simulink model "mono_camera_lane_tracking_with_ros"  (R2019b)
settings: Solver=FixedStepDiscrete  StartTime=0.0  StopTime=inf  FixedStep=Ts  RelTol=1e-3
undefined symbols (not defined in the file): PredictionHorizon, Ts
libraries: robotlib x17, mpcadaslib x1
settings Model: Creator=The MathWorks, Inc.  LastModifiedBy=senoa95
settings DataIOCC: SaveOutput=off  SaveTime=off  ReturnWorkspaceOutputs=off
settings OptimizationCC: DefaultParameterBehavior=Inlined  UseDivisionForNetSlopeComputation=on  GainParamInheritBuiltInType=on  UseFloatMulNetSlope=on  DefaultUnderspecifiedDataType=single  InlineInvariantSignals=on  PassReuseOutputArgsAs=Individual arguments  ZeroExternalMemoryAtStartup=off  ZeroInternalMemoryAtStartup=off  NoFixptDivByZeroProtection=on  EfficientFloat2IntCast=on  LifeSpan=1  OptimizeBlockOrder=speed  DifferentSizesBufferReuse=on  EfficientTunableParamExpr=on
settings DebuggingCC: ParameterPrecisionLossMsg=none  ParameterTunabilityLossMsg=error  PregeneratedLibrarySubsystemCodeDiagnostic=none  ArithmeticOperatorsInVariantConditions=warning
settings HardwareCC: ProdBitPerLong=64  ProdLongLongMode=on  ProdHWDeviceType=Intel->x86-64 (Linux 64)
settings SFSimCC: SimUseLocalCustomCode=off  MATLABDynamicMemAlloc=off
settings RTWCC: SystemTargetFile=ert.tlc  TemplateMakefile=ert_default_tmf  GenerateReport=on  RTWUseLocalCustomCode=off  BuildConfiguration=Faster Runs  IncludeHyperlinkInReport=on  LaunchReport=on  TargetLang=C++  GenerateTraceInfo=on  GenerateTraceReport=on  GenerateTraceReportSl=on  GenerateTraceReportSf=on  GenerateTraceReportEml=on
settings CodeAppCC: ForceParamTrailComments=on  IgnoreCustomStorageClasses=off  MaxIdLength=63  OperatorAnnotations=on  SimulinkDataObjDesc=on  SFDataObjDesc=on  CustomSymbolStrGlobalVar=rt$N$M  CustomSymbolStrType=$N$M  CustomSymbolStrFcn=$N$M$F  CustomSymbolStrMacro=$N$M  InsertBlockDesc=on
settings ERTTargetCC: TargetLangStandard=C++03 (ISO)  GenerateSampleERTMain=on  IncludeMdlTerminateFcn=off  CombineSignalStateStructs=on  SupportAbsoluteTime=off  MultiInstanceERTCode=on  CodeInterfacePackaging=C++ class  SupportComplex=off  SupportNonInlinedSFcns=on  InlinedParameterPlacement=NonHierarchical  RootIOFormat=Structure reference  ERTCustomFileTemplate=example_file_process.tlc

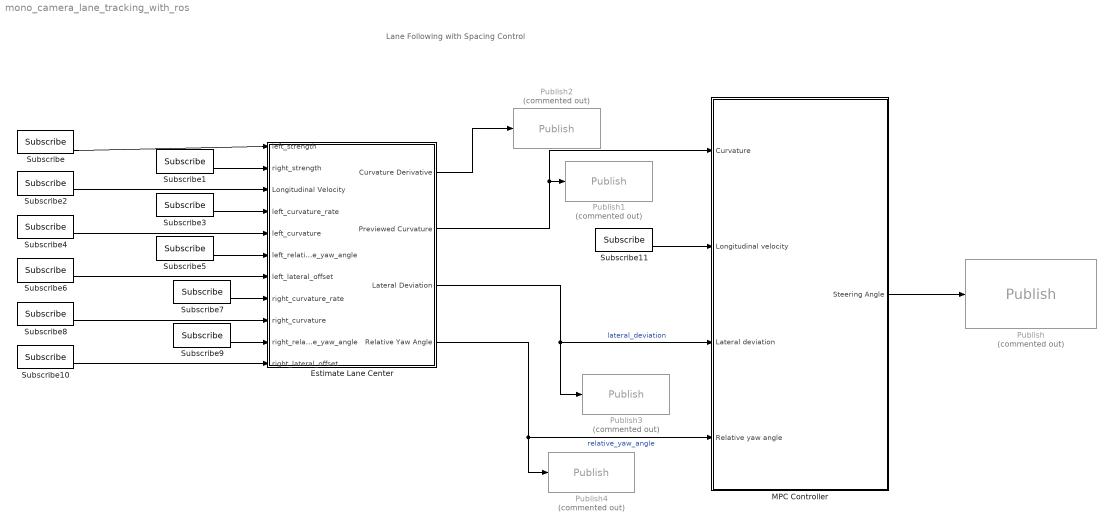
== system mono_camera_lane_tracking_with_ros ==
  note: Lane Following with Spacing Control
  Estimate Lane Center : Subsystem  TreatAsAtomicUnit=on  VariantControl=v2
      settings: RTWFileNameOpts=Use function name
  "MPC Controller " : Subsystem
  Publish : robotlib/Publish  Commented=on  topicSource=Specify your own  topic=/steering_angle  messageType=geometry_msgs/Point  messageQueueLength=1
      settings: SourceProductName=ROS Toolbox
  Publish1 : robotlib/Publish  Commented=on  topicSource=Specify your own  topic=/lane/center/curvature  messageType=std_msgs/Int32  messageQueueLength=1
      settings: SourceProductName=ROS Toolbox
  Publish2 : robotlib/Publish  Commented=on  topicSource=Specify your own  topic=/lane/center/curvature_derivative  messageType=std_msgs/Int32  messageQueueLength=1
      settings: SourceProductName=ROS Toolbox
  Publish3 : robotlib/Publish  Commented=on  topicSource=Specify your own  topic=/lane/center/lateral_deviation  messageType=std_msgs/Int32  messageQueueLength=1
      settings: SourceProductName=ROS Toolbox
  Publish4 : robotlib/Publish  Commented=on  topicSource=Specify your own  topic=/lane/center/lateral_deviation  messageType=std_msgs/Int32  messageQueueLength=1
      settings: SourceProductName=ROS Toolbox
  Subscribe : robotlib/Subscribe  topicSource=Specify your own  topic=/lanes/left/strength  messageType=std_msgs/Int32  sampleTime=-1  messageQueueLength=1
      settings: SourceProductName=ROS Toolbox
  Subscribe1 : robotlib/Subscribe  topicSource=Specify your own  topic=/lanes/left/strength  messageType=std_msgs/Int32  sampleTime=-1  messageQueueLength=1
      settings: SourceProductName=ROS Toolbox
  Subscribe10 : robotlib/Subscribe  topicSource=Specify your own  topic=/lanes/right/lateral_offset  messageType=std_msgs/Int32  sampleTime=-1  messageQueueLength=1
      settings: SourceProductName=ROS Toolbox
  Subscribe11 : robotlib/Subscribe  topicSource=Specify your own  topic=/turtle_velocity  messageType=std_msgs/Int32  sampleTime=-1  messageQueueLength=1
      settings: SourceProductName=ROS Toolbox
  Subscribe2 : robotlib/Subscribe  topicSource=Specify your own  topic=/turtle_velocity  messageType=std_msgs/Int32  sampleTime=-1  messageQueueLength=1
      settings: SourceProductName=ROS Toolbox
  Subscribe3 : robotlib/Subscribe  topicSource=Specify your own  topic=/lanes/left/curvature_rate  messageType=std_msgs/Int32  sampleTime=-1  messageQueueLength=1
      settings: SourceProductName=ROS Toolbox
  Subscribe4 : robotlib/Subscribe  topicSource=Specify your own  topic=/lanes/left/curvature  messageType=std_msgs/Int32  sampleTime=-1  messageQueueLength=1
      settings: SourceProductName=ROS Toolbox
  Subscribe5 : robotlib/Subscribe  topicSource=Specify your own  topic=/lanes/left/relative_yaw_angle  messageType=std_msgs/Int32  sampleTime=-1  messageQueueLength=1
      settings: SourceProductName=ROS Toolbox
  Subscribe6 : robotlib/Subscribe  topicSource=Specify your own  topic=/lanes/left/lateral_offset  messageType=std_msgs/Int32  sampleTime=-1  messageQueueLength=1
      settings: SourceProductName=ROS Toolbox
  Subscribe7 : robotlib/Subscribe  topicSource=Specify your own  topic=/lanes/right/curvature_rate  messageType=std_msgs/Int32  sampleTime=-1  messageQueueLength=1
      settings: SourceProductName=ROS Toolbox
  Subscribe8 : robotlib/Subscribe  topicSource=Specify your own  topic=/lanes/right/curvature  messageType=std_msgs/Int32  sampleTime=-1  messageQueueLength=1
      settings: SourceProductName=ROS Toolbox
  Subscribe9 : robotlib/Subscribe  topicSource=Specify your own  topic=/lanes/right/relative_yaw_angle  messageType=std_msgs/Int32  sampleTime=-1  messageQueueLength=1
      settings: SourceProductName=ROS Toolbox
  wires:
  Subscribe11/2 -> "MPC Controller "/2(Longitudinal velocity)
  Estimate Lane Center/2(Previewed Curvature) -> "MPC Controller "/1(Curvature), Publish1/1
  "MPC Controller "/1(Steering Angle) -> Publish/1
  Estimate Lane Center/3(Lateral Deviation) -> Publish3/1, "MPC Controller "/3(Lateral deviation)  "lateral_deviation"
  Estimate Lane Center/4(Relative Yaw Angle) -> Publish4/1, "MPC Controller "/4(Relative yaw angle)  "relative_yaw_angle"
  Subscribe2/2 -> Estimate Lane Center/3(Longitudinal Velocity)
  Subscribe/2 -> Estimate Lane Center/1(left_strength)
  Subscribe1/2 -> Estimate Lane Center/2(right_strength)
  Subscribe3/2 -> Estimate Lane Center/4(left_curvature_rate)
  Subscribe4/2 -> Estimate Lane Center/5(left_curvature)
  Subscribe6/2 -> Estimate Lane Center/7(left_lateral_offset)
  Subscribe5/2 -> Estimate Lane Center/6(left_relative_yaw_angle)
  Subscribe7/2 -> Estimate Lane Center/8(right_curvature_rate)
  Subscribe8/2 -> Estimate Lane Center/9(right_curvature)
  Subscribe9/2 -> Estimate Lane Center/10(right_relative_yaw_angle)
  Subscribe10/2 -> Estimate Lane Center/11(right_lateral_offset)
  Estimate Lane Center/1(Curvature Derivative) -> Publish2/1

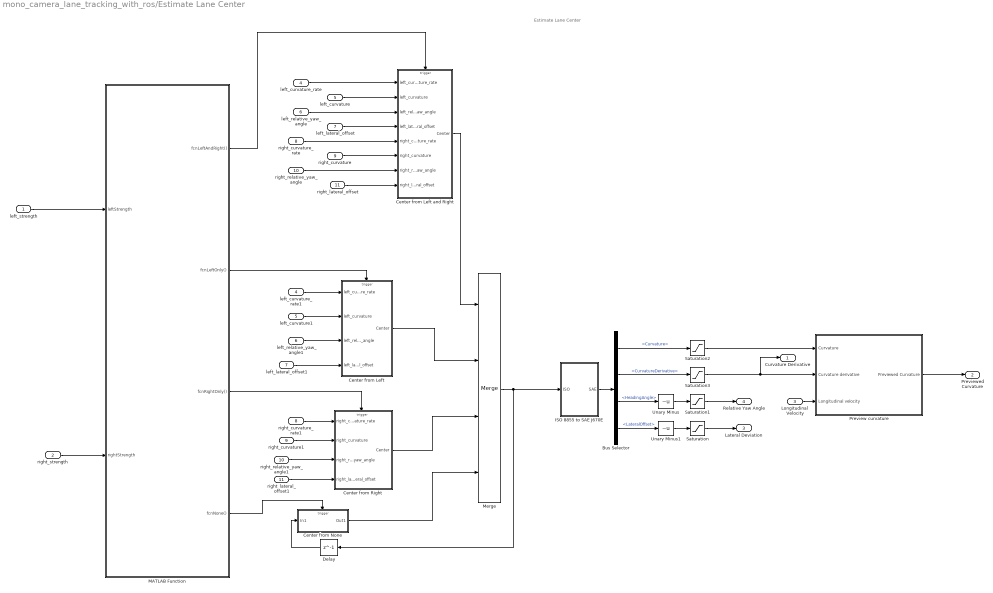
== system mono_camera_lane_tracking_with_ros/Estimate Lane Center ==
  note: Estimate Lane Center
  left_strength : Inport
  right_strength : Inport  Port=2
  Longitudinal Velocity : Inport  Port=3
  left_curvature_rate : Inport  Port=4
  left_curvature : Inport  Port=5
  left_relative_yaw_angle : Inport  Port=6
  left_lateral_offset : Inport  Port=7
  right_curvature_rate : Inport  Port=8
  right_curvature : Inport  Port=9
  right_relative_yaw_angle : Inport  Port=10
  right_lateral_offset : Inport  Port=11
  Bus Selector : BusSelector  OutputSignals=Curvature,CurvatureDerivative,HeadingAngle,LateralOffset
  Center from Left : Subsystem  TreatAsAtomicUnit=on
  Center from Left and Right : Subsystem  TreatAsAtomicUnit=on
  Center from None : Subsystem  TreatAsAtomicUnit=on
  Center from Right : Subsystem  TreatAsAtomicUnit=on
  Delay : Delay  DelayLength=1
  ISO 8855 to SAE J670E : Subsystem
  MATLAB Function : MATLAB Function  TreatAsAtomicUnit=on
  Merge : Merge  Inputs=4
  Preview curvature : Subsystem
  Saturation : Saturate
  Saturation1 : Saturate  UpperLimit=0.6  LowerLimit=-0.6
  Saturation2 : Saturate  UpperLimit=0.15  LowerLimit=-0.15
  Saturation3 : Saturate  UpperLimit=0.06  LowerLimit=-0.06
  Unary Minus : UnaryMinus
  Unary Minus1 : UnaryMinus
  left_curvature1 : InportShadow  Port=5
  left_curvature_rate1 : InportShadow  Port=4
  left_lateral_offset1 : InportShadow  Port=7
  left_relative_yaw_angle1 : InportShadow  Port=6
  right_curvature1 : InportShadow  Port=9
  right_curvature_rate1 : InportShadow  Port=8
  right_lateral_offset1 : InportShadow  Port=11
  right_relative_yaw_angle1 : InportShadow  Port=10
  Curvature Derivative : Outport  OutDataTypeStr=int32
  Previewed Curvature : Outport  Port=2  OutDataTypeStr=int32  VectorParamsAs1DForOutWhenUnconnected=off
  Lateral Deviation : Outport  Port=3  OutDataTypeStr=int32  VectorParamsAs1DForOutWhenUnconnected=off
  Relative Yaw Angle : Outport  Port=4  OutDataTypeStr=int32  VectorParamsAs1DForOutWhenUnconnected=off
  wires:
  Center from Right/1(Center) -> Merge/3
  MATLAB Function/2(fcnLeftOnly()) -> Center from Left/Trigger
  Center from None/1(Out1) -> Merge/4
  MATLAB Function/1(fcnLeftAndRight()) -> Center from Left and Right/Trigger
  Delay/1 -> Center from None/1(In1)
  Center from Left and Right/1(Center) -> Merge/1
  MATLAB Function/3(fcnRightOnly()) -> Center from Right/Trigger
  MATLAB Function/4(fcnNone()) -> Center from None/Trigger
  Center from Left/1(Center) -> Merge/2
  Merge/1 -> ISO 8855 to SAE J670E/1(ISO), Delay/1
  Saturation3/1 -> Curvature Derivative/1, Preview curvature/2(Curvature derivative)
  Saturation2/1 -> Preview curvature/1(Curvature)
  Saturation1/1 -> Relative Yaw Angle/1
  Saturation/1 -> Lateral Deviation/1
  Unary Minus/1 -> Saturation1/1
  Preview curvature/1(Previewed Curvature) -> Previewed Curvature/1
  Longitudinal Velocity/1 -> Preview curvature/3(Longitudinal velocity)
  Bus Selector/2 -> Saturation3/1  "<CurvatureDerivative>"
  Bus Selector/1 -> Saturation2/1  "<Curvature>"
  Unary Minus1/1 -> Saturation/1
  Bus Selector/4 -> Unary Minus1/1  "<LateralOffset>"
  Bus Selector/3 -> Unary Minus/1  "<HeadingAngle>"
  ISO 8855 to SAE J670E/1(SAE) -> Bus Selector/1
  left_strength/1 -> MATLAB Function/1(leftStrength)
  right_strength/1 -> MATLAB Function/2(rightStrength)
  left_curvature_rate/1 -> Center from Left and Right/1(left_curvature_rate)
  right_relative_yaw_angle/1 -> Center from Left and Right/7(right_relative_yaw_angle)
  right_lateral_offset/1 -> Center from Left and Right/8(right_lateral_offset)
  left_lateral_offset/1 -> Center from Left and Right/4(left_lateral_offset)
  left_curvature/1 -> Center from Left and Right/2(left_curvature)
  left_relative_yaw_angle/1 -> Center from Left and Right/3(left_relative_yaw_angle)
  right_curvature_rate/1 -> Center from Left and Right/5(right_curvature_rate)
  right_curvature/1 -> Center from Left and Right/6(right_curvature)
  left_curvature_rate1/1 -> Center from Left/1(left_curvature_rate)
  left_curvature1/1 -> Center from Left/2(left_curvature)
  left_relative_yaw_angle1/1 -> Center from Left/3(left_relative_yaw_angle)
  left_lateral_offset1/1 -> Center from Left/4(left_lateral_offset)
  right_curvature_rate1/1 -> Center from Right/1(right_curvature_rate)
  right_curvature1/1 -> Center from Right/2(right_curvature)
  right_relative_yaw_angle1/1 -> Center from Right/3(right_relative_yaw_angle)
  right_lateral_offset1/1 -> Center from Right/4(right_lateral_offset)

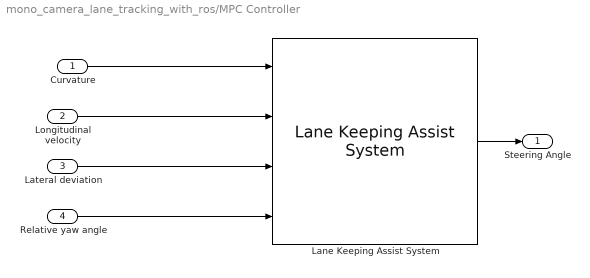
== system mono_camera_lane_tracking_with_ros/MPC Controller  ==
  Curvature : Inport
  Longitudinal velocity : Inport  Port=2
  Lateral deviation : Inport  Port=3
  Relative yaw angle : Inport  Port=4
  Lane Keeping Assist System : mpcadaslib/Lane Keeping Assist System  ModelType=Use vehicle parameters  VehicleMass=1575  VehicleYawInertia=2875  LengthToFront=1.2  LengthToRear=1.6  FrontTireStiffness=19000  RearTireStiffness=33000  EgoModelMatrixA=[-4.4021 ,-12.4603;1.3913,-5.1868]  EgoModelMatrixB=[24.1270;15.8609]  EgoModelMatrixC=[1,0;0,1]  InitialLongVel=15  TransportLag=0  MinSteering=-0.26  umin_ext=off  MaxSteering=0.26  umax_ext=off  Ts=0.1  PredictionHorizon=10  ControllerBehavior=0.5  suboptimal=off  maxiter=10  datatypeopt=double  optmode=off  trackmode=off
      settings: SourceProductName=Model Predictive Control Toolbox  SourceProductBaseCode=MP
  Steering Angle : Outport  OutDataTypeStr=int32  VectorParamsAs1DForOutWhenUnconnected=off
  wires:
  Lane Keeping Assist System/1 -> Steering Angle/1
  Curvature/1 -> Lane Keeping Assist System/1
  Longitudinal velocity/1 -> Lane Keeping Assist System/2
  Lateral deviation/1 -> Lane Keeping Assist System/3
  Relative yaw angle/1 -> Lane Keeping Assist System/4

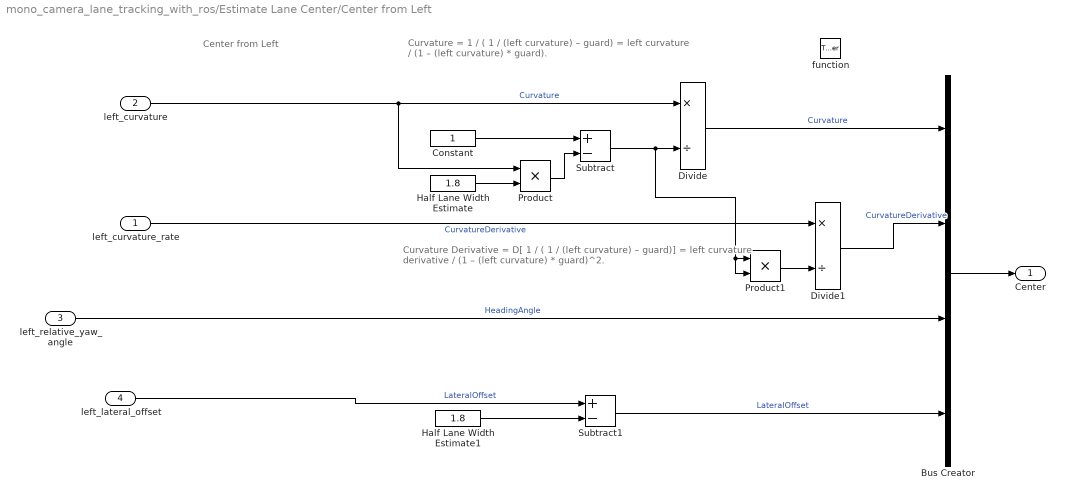
== system mono_camera_lane_tracking_with_ros/Estimate Lane Center/Center from Left ==
  note: Curvature Derivative
      | = D[ 1 / ( 1 / (left curvature) – guard)]
      | = left curvature derivative / (1 – (left curvature) * guard)^2.
  note: Center from Left
  note: Curvature
      | = 1 / ( 1 / (left curvature) – guard)
      | = left curvature / (1 – (left curvature) * guard).
  left_curvature_rate : Inport
  left_curvature : Inport  Port=2
  left_relative_yaw_angle : Inport  Port=3
  left_lateral_offset : Inport  Port=4
  function : TriggerPort  TriggerType=function-call  VariantControl=Variant
  Bus Creator : BusCreator  Inputs=4
  Constant : Constant  OutDataTypeStr=Inherit: Inherit via back propagation
  Divide : Product  Inputs=*/
  Divide1 : Product  Inputs=*/
  Half Lane Width Estimate : Constant  Value=1.8  OutDataTypeStr=Inherit: Inherit via back propagation
  Half Lane Width Estimate1 : Constant  Value=1.8  OutDataTypeStr=Inherit: Inherit via back propagation
  Product : Product
  Product1 : Product
  Subtract : Sum  Inputs=+-
  Subtract1 : Sum  Inputs=+-
  Center : Outport  VectorParamsAs1DForOutWhenUnconnected=off
  wires:
  Product/1 -> Subtract/2
  Half Lane Width Estimate1/1 -> Subtract1/2
  left_lateral_offset/1 -> Subtract1/1  "LateralOffset"
  Product1/1 -> Divide1/2
  left_curvature_rate/1 -> Divide1/1  "CurvatureDerivative"
  Constant/1 -> Subtract/1
  Half Lane Width Estimate/1 -> Product/2
  Subtract/1 -> Divide/2, Product1/1, Product1/2
  left_curvature/1 -> Divide/1, Product/1  "Curvature"
  Subtract1/1 -> Bus Creator/4  "LateralOffset"
  left_relative_yaw_angle/1 -> Bus Creator/3  "HeadingAngle"
  Divide/1 -> Bus Creator/1  "Curvature"
  Divide1/1 -> Bus Creator/2  "CurvatureDerivative"
  Bus Creator/1 -> Center/1

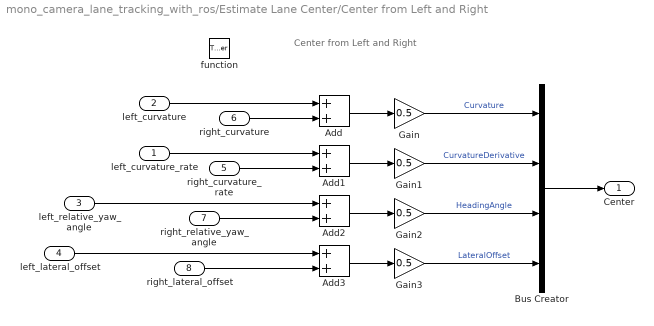
== system mono_camera_lane_tracking_with_ros/Estimate Lane Center/Center from Left and Right ==
  note: Center from Left and Right
  left_curvature_rate : Inport
  left_curvature : Inport  Port=2
  left_relative_yaw_angle : Inport  Port=3
  left_lateral_offset : Inport  Port=4
  right_curvature_rate : Inport  Port=5
  right_curvature : Inport  Port=6
  right_relative_yaw_angle : Inport  Port=7
  right_lateral_offset : Inport  Port=8
  function : TriggerPort  TriggerType=function-call  VariantControl=Variant
  Add{,1..3} (4 alike) : Sum
  Bus Creator : BusCreator  Inputs=4
  Gain{,1..3} (4 alike) : Gain  Gain=0.5
  Center : Outport  VectorParamsAs1DForOutWhenUnconnected=off
  wires:
  left_lateral_offset/1 -> Add3/1
  right_lateral_offset/1 -> Add3/2
  right_relative_yaw_angle/1 -> Add2/2
  left_relative_yaw_angle/1 -> Add2/1
  right_curvature_rate/1 -> Add1/2
  left_curvature_rate/1 -> Add1/1
  left_curvature/1 -> Add/1
  Bus Creator/1 -> Center/1
  Gain3/1 -> Bus Creator/4  "LateralOffset"
  Add3/1 -> Gain3/1
  Gain2/1 -> Bus Creator/3  "HeadingAngle"
  Add2/1 -> Gain2/1
  Gain1/1 -> Bus Creator/2  "CurvatureDerivative"
  Add1/1 -> Gain1/1
  Gain/1 -> Bus Creator/1  "Curvature"
  Add/1 -> Gain/1
  right_curvature/1 -> Add/2

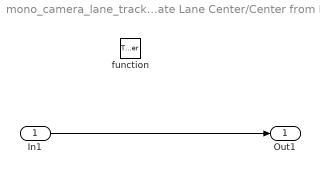
== system mono_camera_lane_tracking_with_ros/Estimate Lane Center/Center from None ==
  In1 : Inport
  function : TriggerPort  TriggerType=function-call  VariantControl=Variant
  Out1 : Outport  VectorParamsAs1DForOutWhenUnconnected=off
  wires:
  In1/1 -> Out1/1

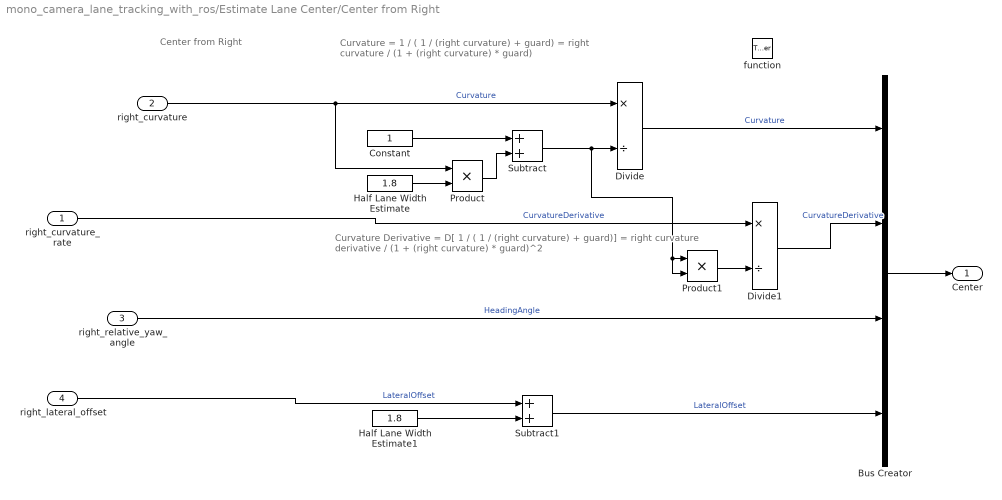
== system mono_camera_lane_tracking_with_ros/Estimate Lane Center/Center from Right ==
  note: Curvature Derivative
      | = D[ 1 / ( 1 / (right curvature) + guard)]
      | = right curvature derivative / (1 + (right curvature) * guard)^2
  note: Curvature
      | = 1 / ( 1 / (right curvature) + guard)
      | = right curvature / (1 + (right curvature) * guard)
  note: Center from Right
  right_curvature_rate : Inport
  right_curvature : Inport  Port=2
  right_relative_yaw_angle : Inport  Port=3
  right_lateral_offset : Inport  Port=4
  function : TriggerPort  TriggerType=function-call  VariantControl=Variant
  Bus Creator : BusCreator  Inputs=4
  Constant : Constant  OutDataTypeStr=Inherit: Inherit via back propagation
  Divide : Product  Inputs=*/
  Divide1 : Product  Inputs=*/
  Half Lane Width Estimate : Constant  Value=1.8  OutDataTypeStr=Inherit: Inherit via back propagation
  Half Lane Width Estimate1 : Constant  Value=1.8  OutDataTypeStr=Inherit: Inherit via back propagation
  Product : Product
  Product1 : Product
  Subtract : Sum
  Subtract1 : Sum
  Center : Outport  VectorParamsAs1DForOutWhenUnconnected=off
  wires:
  Half Lane Width Estimate/1 -> Product/2
  Product/1 -> Subtract/2
  Constant/1 -> Subtract/1
  Subtract/1 -> Divide/2, Product1/1, Product1/2
  right_curvature/1 -> Divide/1, Product/1  "Curvature"
  Bus Creator/1 -> Center/1
  Subtract1/1 -> Bus Creator/4  "LateralOffset"
  Divide/1 -> Bus Creator/1  "Curvature"
  right_lateral_offset/1 -> Subtract1/1  "LateralOffset"
  Half Lane Width Estimate1/1 -> Subtract1/2
  right_relative_yaw_angle/1 -> Bus Creator/3  "HeadingAngle"
  Product1/1 -> Divide1/2
  Divide1/1 -> Bus Creator/2  "CurvatureDerivative"
  right_curvature_rate/1 -> Divide1/1  "CurvatureDerivative"

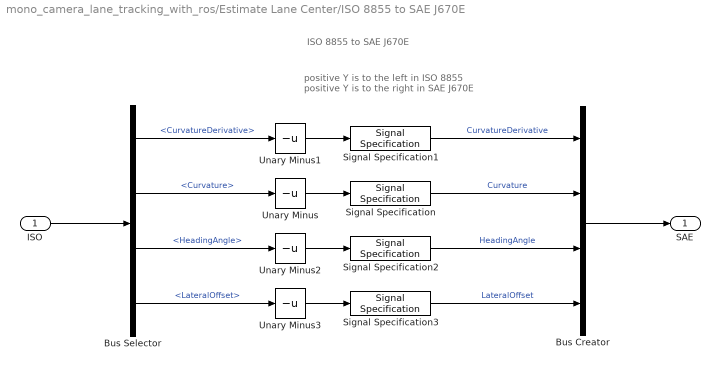
== system mono_camera_lane_tracking_with_ros/Estimate Lane Center/ISO 8855 to SAE J670E ==
  note: positive Y is to the left in ISO 8855
      | positive Y is to the right in SAE J670E
  note: ISO 8855 to SAE J670E
  ISO : Inport
  Bus Creator : BusCreator  Inputs=4
  Bus Selector : BusSelector  OutputSignals=CurvatureDerivative,Curvature,HeadingAngle,LateralOffset
  Signal Specification : SignalSpecification  Unit=1/m^2
  Signal Specification1 : SignalSpecification  Unit=1/m
  Signal Specification2 : SignalSpecification  Unit=rad
  Signal Specification3 : SignalSpecification  Unit=m
  Unary Minus{,1..3} (4 alike) : UnaryMinus
  SAE : Outport  VectorParamsAs1DForOutWhenUnconnected=off
  wires:
  ISO/1 -> Bus Selector/1
  Bus Selector/2 -> Unary Minus/1  "<Curvature>"
  Bus Selector/1 -> Unary Minus1/1  "<CurvatureDerivative>"
  Bus Selector/3 -> Unary Minus2/1  "<HeadingAngle>"
  Bus Selector/4 -> Unary Minus3/1  "<LateralOffset>"
  Bus Creator/1 -> SAE/1
  Signal Specification/1 -> Bus Creator/2  "Curvature"
  Unary Minus1/1 -> Signal Specification1/1
  Unary Minus2/1 -> Signal Specification2/1
  Unary Minus3/1 -> Signal Specification3/1
  Unary Minus/1 -> Signal Specification/1
  Signal Specification1/1 -> Bus Creator/1  "CurvatureDerivative"
  Signal Specification2/1 -> Bus Creator/3  "HeadingAngle"
  Signal Specification3/1 -> Bus Creator/4  "LateralOffset"

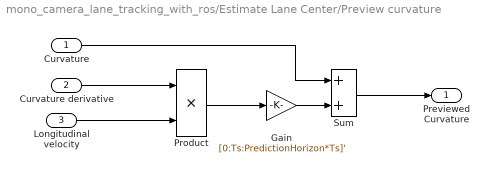
== system mono_camera_lane_tracking_with_ros/Estimate Lane Center/Preview curvature ==
  Curvature : Inport
  Curvature derivative : Inport  Port=2
  Longitudinal velocity : Inport  Port=3
  Gain : Gain  Gain=[0:Ts:PredictionHorizon*Ts]'
  Product : Product
  Sum : Sum
  Previewed Curvature : Outport  VectorParamsAs1DForOutWhenUnconnected=off
  wires:
  Sum/1 -> Previewed Curvature/1
  Curvature/1 -> Sum/1
  Gain/1 -> Sum/2
  Product/1 -> Gain/1
  Longitudinal velocity/1 -> Product/2
  Curvature derivative/1 -> Product/1

== matlab function mono_camera_lane_tracking_with_ros/Estimate Lane Center/MATLAB Function ==
  data: leftStrength input; rightStrength input
  events: fcnLeftAndRight output FUNCTION_CALL_EVENT; fcnLeftOnly output FUNCTION_CALL_EVENT; fcnRightOnly output FUNCTION_CALL_EVENT; fcnNone output FUNCTION_CALL_EVENT
function fcn(leftStrength,rightStrength)

% leftStrength  = lanes.Left.Strength;
% rightStrength = lanes.Right.Strength;

if (leftStrength > 0) && (rightStrength > 0)
   fcnLeftAndRight();
   
elseif leftStrength > 0
    fcnLeftOnly();
    
elseif rightStrength > 0
    fcnRightOnly();
    
else
    fcnNone();
end
